simulink model "ruido"  (R2022a)
settings: Solver=VariableStepAuto  StartTime=0.0  StopTime=inf  RelTol=1e-3
undefined symbols (not defined in the file or in its folder): none, Rec, SDTV, videoinput
libraries: visionconversions x2, imaqlib x1
settings Model: Creator=misog  LastModifiedBy=misog

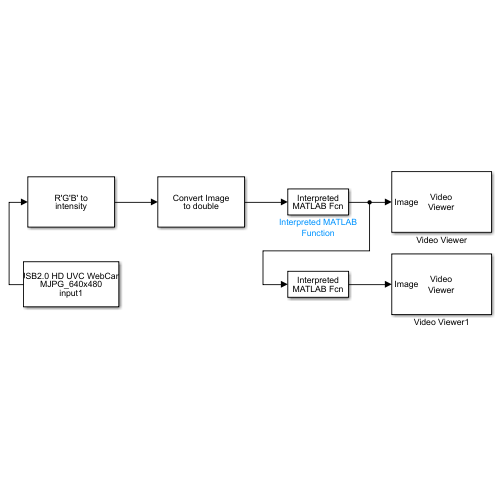
[thumbnail: Simulink's stored preview of the top-level diagram]
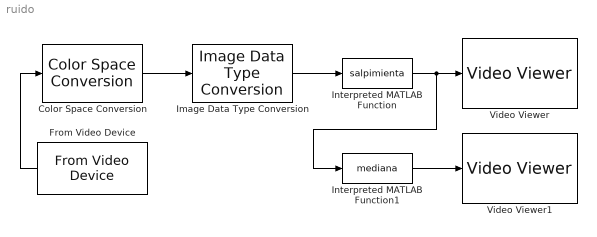
== system ruido ==
  Color Space Conversion : visionconversions/Color Space  Conversion  conversion=Obsolete  conversionActive=R'G'B' to intensity  wp_str=D65  rec=Rec. 601 (SDTV)  sys=1125/60/2:1  imagePorts=One multidimensional signal
  From Video Device : imaqlib/From Video Device  DeviceMenu=winvideo 1 (USB2.0 HD UVC WebCam)  Device=winvideo 1 (USB2.0 HD UVC WebCam)  ObjConstructor=videoinput('winvideo', 1)  VideoFormatMenu=MJPG_640x480  VideoFormat=MJPG_640x480  VideoSource=input1  ROIPosition=[0 0 480 640]  EnableHWTrigger=off  TriggerConfiguration=none/none  SampleTime=1/30  OutputPortsMode=One multidimensional signal  DataType=single  CanDoHWTrigger=no  ReturnedColorSpace=rgb  BlockHandle=4.0002  ROIWidth=640  ROIHeight=480  ROIColumn=0  ROIRow=0  EngXMLPath=C:\Program Files\MATLAB\R2022a\toolbox\imaq\imaq\private  DevXMLPath=C:\ProgramData\MATLAB\SupportPackages\R2022a\toolbox\imaq\supportpackages\genericvideo\adaptor\win64  EngLibPath=C:\Program Files\MATLAB\R2022a\toolbox\imaq\imaqblks\imaqmex\win64  ColorSpace=rgb  BayerSensorAlignment=grbg  ImaqMode=off
  Image Data Type Conversion : visionconversions/Image Data Type Conversion  outDT=double  isSigned=on  wordLen=16  numFracBits=0
      settings: SourceProductBaseCode=VP
  Interpreted MATLAB Function : MATLABFcn  MATLABFcn=salpimienta  Output1D=off
  Interpreted MATLAB Function1 : MATLABFcn  MATLABFcn=mediana  Output1D=off
  Video Viewer : VideoViewer  FigPos=[2 1077 958 969]
  Video Viewer1 : VideoViewer  FigPos=[962 1077 958 969]
  wires:
  From Video Device/1 -> Color Space Conversion/1
  Color Space Conversion/1 -> Image Data Type Conversion/1
  Image Data Type Conversion/1 -> Interpreted MATLAB Function/1
  Interpreted MATLAB Function/1 -> Interpreted MATLAB Function1/1, Video Viewer/1
  Interpreted MATLAB Function1/1 -> Video Viewer1/1
